simulink model "ECU_Arch"  (R2022b)
settings: Solver=FixedStepDiscrete  StartTime=0.0  StopTime=10.0  RelTol=1e-3
InitFcn:
  | mbd_mpc_consistency_checks(bdroot(gcs));
model workspace (MAT data in the model file):
  AlignmentIdRef = Simulink.Parameter
  AlignmentIdRef.Value = 0.3
  AlignmentIdRef.Description = 'The required IdRef ( which applaies a voltage vector) to aligne the rotor to detect the encoder or resolver offset'
  AlignmentIdRef.DataType = 'single'
  AlignmentIdRef.Min = 0.1
  AlignmentIdRef.Max = 100
  AlignmentIdRef.DocUnits = 'A'
  AlignmentIdRef.Complexity = 'real'
  AlignmentIdRef.Dimensions = [1 1]
  Alignment_ReqTime_sec = Simulink.Parameter
  Alignment_ReqTime_sec.Value = 3
  Alignment_ReqTime_sec.DataType = 'single'
  Alignment_ReqTime_sec.Min = 0
  Alignment_ReqTime_sec.Max = 20
  Alignment_ReqTime_sec.Complexity = 'real'
  Alignment_ReqTime_sec.Dimensions = [1 1]
  AliveCounterStartGD = Simulink.Signal
  AliveCounterStartGD.Description = 'Alive counter to check the length of the Init of GateDriver'
  AliveCounterStartGD.DataType = 'single'
  AliveCounterStartGD.Min = -1000000
  AliveCounterStartGD.Max = 1000000
  AliveCounterStartGD.DocUnits = '-'
  AliveCounterStartGD.Dimensions = -1
  AliveCounterStartGD.DimensionsMode = 'auto'
  AliveCounterStartGD.Complexity = 'auto'
  AliveCounterStartGD.SampleTime = -1
  AliveCounterStartGD.SamplingMode = 'auto'
  AliveCounterStartGD.InitialValue = '0'
  AngleChangeDir = Simulink.Parameter
  AngleChangeDir.Value = 1
  AngleChangeDir.Description = 'It can be used to change the direction of the postion signal, but by default = 1'
  AngleChangeDir.DataType = 'single'
  AngleChangeDir.Min = -1
  AngleChangeDir.Max = 1
  AngleChangeDir.Complexity = 'real'
  AngleChangeDir.Dimensions = [1 1]
  C_LST = 0.0001
  CtrlMode = Simulink.Parameter
  CtrlMode.Value = 1
  CtrlMode.DataType = 'single'
  CtrlMode.Min = 0
  CtrlMode.Max = 1
  CtrlMode.Complexity = 'real'
  CtrlMode.Dimensions = [1 1]
  DelayTimeAfterOL_sec = Simulink.Parameter
  DelayTimeAfterOL_sec.Value = 5
  DelayTimeAfterOL_sec.DataType = 'single'
  DelayTimeAfterOL_sec.Min = 0
  DelayTimeAfterOL_sec.Max = 100
  DelayTimeAfterOL_sec.Complexity = 'real'
  DelayTimeAfterOL_sec.Dimensions = [1 1]
  DisablePWM = Simulink.Parameter
  DisablePWM.Value = 0
  DisablePWM.Description = 'Disable the PWM during the Rotor Offset Calibration'
  DisablePWM.DataType = 'single'
  DisablePWM.Min = 0
  DisablePWM.Max = 1
  DisablePWM.Complexity = 'real'
  DisablePWM.Dimensions = [1 1]
  DisablePWM_Selector = Simulink.Parameter
  DisablePWM_Selector.Value = 0
  DisablePWM_Selector.Description = 'select either without or with Disable the PWM during the Rotor Offset Calibration'
  DisablePWM_Selector.DataType = 'uint8'
  DisablePWM_Selector.Min = 0
  DisablePWM_Selector.Max = 1
  DisablePWM_Selector.DocUnits = '-'
  DisablePWM_Selector.Complexity = 'real'
  DisablePWM_Selector.Dimensions = [1 1]
  ExecutionTimeFastLoop_FOC = Simulink.Parameter
  ExecutionTimeFastLoop_FOC.Value = 0
  ExecutionTimeFastLoop_FOC.Description = 'to measure the execution time of the subsystem'
  ExecutionTimeFastLoop_FOC.DataType = 'single'
  ExecutionTimeFastLoop_FOC.Min = 0
  ExecutionTimeFastLoop_FOC.Max = 1000000
  ExecutionTimeFastLoop_FOC.Complexity = 'real'
  ExecutionTimeFastLoop_FOC.Dimensions = [1 1]
  IDcFilterConst = Simulink.Parameter
  IDcFilterConst.Value = 0.001
  IDcFilterConst.Description = 'Time constant of the FIR IDc current filter '
  IDcFilterConst.DataType = 'single'
  IDcFilterConst.Min = 0
  IDcFilterConst.Max = 1
  IDcFilterConst.Complexity = 'real'
  IDcFilterConst.Dimensions = [1 1]
  IDcFilterSelector = Simulink.Parameter
  IDcFilterSelector.Value = 0
  IDcFilterSelector.Description = 'Switch to select one of the applied IDc current filter '
  IDcFilterSelector.DataType = 'uint16'
  IDcFilterSelector.Min = 0
  IDcFilterSelector.Max = 1
  IDcFilterSelector.Complexity = 'real'
  IDcFilterSelector.Dimensions = [1 1]
  IDcOvercurrent = Simulink.Parameter
  IDcOvercurrent.Value = 5
  IDcOvercurrent.Description = 'value of the overcurrent'
  IDcOvercurrent.DataType = 'single'
  IDcOvercurrent.Min = 0.1
  IDcOvercurrent.Max = 100
  IDcOvercurrent.DocUnits = 'A'
  IDcOvercurrent.Complexity = 'real'
  IDcOvercurrent.Dimensions = [1 1]
  IDcOvercurrentAlignment = Simulink.Parameter
  IDcOvercurrentAlignment.Value = 6
  IDcOvercurrentAlignment.Description = 'Idc overcurrent limit during rotor alignment to detect the encoder or resolver offset'
  IDcOvercurrentAlignment.DataType = 'single'
  IDcOvercurrentAlignment.Min = 0.1
  IDcOvercurrentAlignment.Max = 100
  IDcOvercurrentAlignment.DocUnits = 'A'
  IDcOvercurrentAlignment.Complexity = 'real'
  IDcOvercurrentAlignment.Dimensions = [1 1]
  IQ_REF = Simulink.Signal
  IQ_REF.Description = 'The reference iq'
  IQ_REF.DataType = 'single'
  IQ_REF.Min = -100
  IQ_REF.Max = 100
  IQ_REF.DocUnits = 'A'
  IQ_REF.Dimensions = -1
  IQ_REF.DimensionsMode = 'auto'
  IQ_REF.Complexity = 'real'
  IQ_REF.SampleTime = -1
  IQ_REF.SamplingMode = 'auto'
  IQ_REF.InitialValue = '0'
  IQ_REF_MAX = Simulink.Parameter
  IQ_REF_MAX.Value = 2.3
  IQ_REF_MAX.Description = 'Maximum allowed Iq current to limit the output of the speed controller'
  IQ_REF_MAX.DataType = 'single'
  IQ_REF_MAX.Min = -100
  IQ_REF_MAX.Max = 100
  IQ_REF_MAX.DocUnits = 'A'
  IQ_REF_MAX.Complexity = 'real'
  IQ_REF_MAX.Dimensions = [1 1]
  I_MAX = Simulink.Parameter
  I_MAX.Value = 20.625
  I_MAX.Description = 'Maximum current used for current measurement scaling calibration'
  I_MAX.DataType = 'single'
  I_MAX.Min = -100
  I_MAX.Max = 100
  I_MAX.DocUnits = 'A'
  I_MAX.Complexity = 'real'
  I_MAX.Dimensions = [1 1]
  KiId = Simulink.Parameter
  KiId.Value = 0.5
  KiId.Description = 'proportional parameter Kp of the ID-current controller'
  KiId.DataType = 'single'
  KiId.Min = 0
  KiId.Max = 1000
  KiId.Complexity = 'real'
  KiId.Dimensions = [1 1]
  KiIq = Simulink.Parameter
  KiIq.Value = 0.5
  KiIq.Description = 'proportional parameter Kp of the IQ-current controller'
  KiIq.DataType = 'single'
  KiIq.Min = 0
  KiIq.Max = 1000
  KiIq.Complexity = 'real'
  KiIq.Dimensions = [1 1]
  KiSpd = Simulink.Parameter
  KiSpd.Value = 1
  KiSpd.Description = 'propotinal factor of speed controller'
  KiSpd.DataType = 'single'
  KiSpd.Min = 0
  KiSpd.Max = 1000
  KiSpd.Complexity = 'real'
  KiSpd.Dimensions = [1 1]
  KiSpdOrg = Simulink.Parameter
  KiSpdOrg.Value = 2.2316799098e-05
  KiSpdOrg.Description = 'propotinal factor of speed controller'
  KiSpdOrg.DataType = 'single'
  KiSpdOrg.Min = 0
  KiSpdOrg.Max = 1000
  KiSpdOrg.Complexity = 'real'
  KiSpdOrg.Dimensions = [1 1]
  KpId = Simulink.Parameter
  KpId.Value = 0.3
  KpId.Description = 'proportional parameter Kp of the ID-current controller'
  KpId.DataType = 'single'
  KpId.Min = 0
  KpId.Max = 1000
  KpId.Complexity = 'real'
  KpId.Dimensions = [1 1]
  KpIq = Simulink.Parameter
  KpIq.Value = 0.3
  KpIq.Description = 'proportional parameter Kp of the IQ-current controller'
  KpIq.DataType = 'single'
  KpIq.Min = 0
  KpIq.Max = 1000
  KpIq.Complexity = 'real'
  KpIq.Dimensions = [1 1]
  KpSpd = Simulink.Parameter
  KpSpd.Value = 1.5
  KpSpd.Description = 'propotinal factor of speed controller'
  KpSpd.DataType = 'single'
  KpSpd.Min = 0
  KpSpd.Max = 1000
  KpSpd.Complexity = 'real'
  KpSpd.Dimensions = [1 1]
  KpSpdOrg = Simulink.Parameter
  KpSpdOrg.Value = 0.0142073155617
  KpSpdOrg.Description = 'propotinal factor of speed controller'
  KpSpdOrg.DataType = 'single'
  KpSpdOrg.Min = 0
  KpSpdOrg.Max = 1000
  KpSpdOrg.Complexity = 'real'
  KpSpdOrg.Dimensions = [1 1]
  Low_TQLimit_SpdCtrl = Simulink.Parameter
  Low_TQLimit_SpdCtrl.Value = -0.12
  Low_TQLimit_SpdCtrl.DataType = 'single'
  Low_TQLimit_SpdCtrl.Min = -10
  Low_TQLimit_SpdCtrl.Max = 0
  Low_TQLimit_SpdCtrl.Complexity = 'real'
  Low_TQLimit_SpdCtrl.Dimensions = [1 1]
  Low_TQLimit_TqCtrl = Simulink.Parameter
  Low_TQLimit_TqCtrl.Value = -0.04
  Low_TQLimit_TqCtrl.DataType = 'single'
  Low_TQLimit_TqCtrl.Min = -10
  Low_TQLimit_TqCtrl.Max = 0
  Low_TQLimit_TqCtrl.Complexity = 'real'
  Low_TQLimit_TqCtrl.Dimensions = [1 1]
  MaxSpdLimit = Simulink.Parameter
  MaxSpdLimit.Value = 199
  MaxSpdLimit.Description = 'Maximum Allowed Speed'
  MaxSpdLimit.DataType = 'single'
  MaxSpdLimit.Min = -524
  MaxSpdLimit.Max = 524
  MaxSpdLimit.DocUnits = 'rad/sec'
  MaxSpdLimit.Complexity = 'real'
  MaxSpdLimit.Dimensions = [1 1]
  Nmax = Simulink.Parameter
  Nmax.Value = 6000
  Nmax.Description = 'polpair'
  Nmax.DataType = 'int32'
  Nmax.Min = 1
  Nmax.Max = 20000
  Nmax.DocUnits = '-'
  Nmax.Complexity = 'real'
  Nmax.Dimensions = [1 1]
  OL_IDcOvercurrent = Simulink.Parameter
  OL_IDcOvercurrent.Value = 5.5
  OL_IDcOvercurrent.DataType = 'single'
  OL_IDcOvercurrent.Min = 0
  OL_IDcOvercurrent.Max = 7
  OL_IDcOvercurrent.Complexity = 'real'
  OL_IDcOvercurrent.Dimensions = [1 1]
  OL_ReqTime_sec = Simulink.Parameter
  OL_ReqTime_sec.Value = 1
  OL_ReqTime_sec.DataType = 'single'
  OL_ReqTime_sec.Min = 0
  OL_ReqTime_sec.Max = 20
  OL_ReqTime_sec.Complexity = 'real'
  OL_ReqTime_sec.Dimensions = [1 1]
  OffsetSelector = Simulink.Parameter
  OffsetSelector.Value = 0
  OffsetSelector.Description = 'switch to select the finial rotor offset either add to the actual rotor position or substract from the actual rotor position'
  OffsetSelector.DataType = 'uint8'
  OffsetSelector.Min = 0
  OffsetSelector.Max = 1
  OffsetSelector.Complexity = 'real'
  OffsetSelector.Dimensions = [1 1]
  PISpdControllerSelector = Simulink.Parameter
  PISpdControllerSelector.Value = 0
  PISpdControllerSelector.Description = 'selector to test the correct PI speed controller'
  PISpdControllerSelector.DataType = 'uint8'
  PISpdControllerSelector.Min = 0
  PISpdControllerSelector.Max = 1
  PISpdControllerSelector.Complexity = 'real'
  PISpdControllerSelector.Dimensions = [1 1]
  PMflux = Simulink.Parameter
  PMflux.Value = 0.0064
  PMflux.DataType = 'single'
  PMflux.Min = 0
  PMflux.Max = 10
  PMflux.Complexity = 'real'
  PMflux.Dimensions = [1 1]
  PP = Simulink.Parameter
  PP.Value = 4
  PP.Description = 'polpair'
  PP.DataType = 'int32'
  PP.Min = 1
  PP.Max = 10
  PP.DocUnits = '-'
  PP.Complexity = 'real'
  PP.Dimensions = [1 1]
  PWMDutyCycle_A = Simulink.Signal
  PWMDutyCycle_A.Description = 'Input of the PWM Phase A '
  PWMDutyCycle_A.DataType = 'single'
  PWMDutyCycle_A.Min = -100
  PWMDutyCycle_A.Max = 100
  PWMDutyCycle_A.DocUnits = '-'
  PWMDutyCycle_A.Dimensions = -1
  PWMDutyCycle_A.DimensionsMode = 'auto'
  PWMDutyCycle_A.Complexity = 'real'
  PWMDutyCycle_A.SampleTime = -1
  PWMDutyCycle_A.SamplingMode = 'auto'
  PWMDutyCycle_A.InitialValue = '0'
  PWMDutyCycle_B = Simulink.Signal
  PWMDutyCycle_B.Description = 'Input of the PWM Phase B '
  PWMDutyCycle_B.DataType = 'single'
  PWMDutyCycle_B.Min = -100
  PWMDutyCycle_B.Max = 100
  PWMDutyCycle_B.DocUnits = '-'
  PWMDutyCycle_B.Dimensions = -1
  PWMDutyCycle_B.DimensionsMode = 'auto'
  PWMDutyCycle_B.Complexity = 'real'
  PWMDutyCycle_B.SampleTime = -1
  PWMDutyCycle_B.SamplingMode = 'auto'
  PWMDutyCycle_B.InitialValue = '0'
  PWMDutyCycle_C = Simulink.Signal
  PWMDutyCycle_C.Description = 'Input of the PWM Phase C '
  PWMDutyCycle_C.DataType = 'single'
  PWMDutyCycle_C.Min = -100
  PWMDutyCycle_C.Max = 100
  PWMDutyCycle_C.DocUnits = '-'
  PWMDutyCycle_C.Dimensions = -1
  PWMDutyCycle_C.DimensionsMode = 'auto'
  PWMDutyCycle_C.Complexity = 'real'
  PWMDutyCycle_C.SampleTime = -1
  PWMDutyCycle_C.SamplingMode = 'auto'
  PWMDutyCycle_C.InitialValue = '0'
  PhA_Offset = Simulink.Parameter
  PhA_Offset.Value = 20.625
  PhA_Offset.Description = 'Offset current value of phase A, which used for current calibration'
  PhA_Offset.DataType = 'single'
  PhA_Offset.Min = -100
  PhA_Offset.Max = 100
  PhA_Offset.DocUnits = 'A'
  PhA_Offset.Complexity = 'real'
  PhA_Offset.Dimensions = [1 1]
  PhB_Offset = Simulink.Parameter
  PhB_Offset.Value = 20.625
  PhB_Offset.Description = 'Offset current value of phase B, which used for current calibration'
  PhB_Offset.DataType = 'single'
  PhB_Offset.Min = -100
  PhB_Offset.Max = 100
  PhB_Offset.DocUnits = 'A'
  PhB_Offset.Complexity = 'real'
  PhB_Offset.Dimensions = [1 1]
  RotorOffsetMotor1_Selector = Simulink.Parameter
  RotorOffsetMotor1_Selector.Value = 1
  RotorOffsetMotor1_Selector.Description = 'Feedback when the rotor offset of motor1 is completed '
  RotorOffsetMotor1_Selector.DataType = 'single'
  RotorOffsetMotor1_Selector.Min = 0
  RotorOffsetMotor1_Selector.Max = 1
  RotorOffsetMotor1_Selector.DocUnits = '-'
  RotorOffsetMotor1_Selector.Complexity = 'real'
  RotorOffsetMotor1_Selector.Dimensions = [1 1]
  RotorOffsetMotor2_Selector = Simulink.Parameter
  RotorOffsetMotor2_Selector.Value = 1
  RotorOffsetMotor2_Selector.Description = 'Feedback when the rotor offset of motor2 is completed '
  RotorOffsetMotor2_Selector.DataType = 'single'
  RotorOffsetMotor2_Selector.Min = 0
  RotorOffsetMotor2_Selector.Max = 1
  RotorOffsetMotor2_Selector.DocUnits = '-'
  RotorOffsetMotor2_Selector.Complexity = 'real'
  RotorOffsetMotor2_Selector.Dimensions = [1 1]
  SPEED_CMD = Simulink.Parameter
  SPEED_CMD.Value = 500
  SPEED_CMD.Description = 'Reference speed in rpm'
  SPEED_CMD.DataType = 'single'
  SPEED_CMD.Min = -2200
  SPEED_CMD.Max = 2200
  SPEED_CMD.Complexity = 'real'
  SPEED_CMD.Dimensions = [1 1]
  SPEED_DOWN_INC = Simulink.Parameter
  SPEED_DOWN_INC.Value = 50
  SPEED_DOWN_INC.Description = 'Gain used to decrease the reference speed (SPEED_CMD)using push botton on the MPC5744P board '
  SPEED_DOWN_INC.DataType = 'single'
  SPEED_DOWN_INC.Min = -1000
  SPEED_DOWN_INC.Max = 1000
  SPEED_DOWN_INC.Complexity = 'real'
  SPEED_DOWN_INC.Dimensions = [1 1]
  SPEED_LOOP_CNTR = Simulink.Parameter
  SPEED_LOOP_CNTR.Value = 10
  SPEED_LOOP_CNTR.Description = 'speed loop counter, which used to determine who many current loops are over to recall the speed loop  '
  SPEED_LOOP_CNTR.DataType = 'single'
  SPEED_LOOP_CNTR.Min = -1000
  SPEED_LOOP_CNTR.Max = 1000
  SPEED_LOOP_CNTR.Complexity = 'real'
  SPEED_LOOP_CNTR.Dimensions = [1 1]
  SPEED_UP_INC = Simulink.Parameter
  SPEED_UP_INC.Value = 50
  SPEED_UP_INC.Description = 'Gain used to decrease the reference speed (SPEED_CMD)using push botton on the MPC5744P board '
  SPEED_UP_INC.DataType = 'single'
  SPEED_UP_INC.Min = -1000
  SPEED_UP_INC.Max = 1000
  SPEED_UP_INC.Complexity = 'real'
  SPEED_UP_INC.Dimensions = [1 1]
  S_LST = 0.001
  SpdChangeDir = Simulink.Parameter
  SpdChangeDir.Value = 1
  SpdChangeDir.Description = 'It can be used to change the direction of the speed signal, but by default = 1'
  SpdChangeDir.DataType = 'single'
  SpdChangeDir.Min = -1
  SpdChangeDir.Max = 1
  SpdChangeDir.Complexity = 'real'
  SpdChangeDir.Dimensions = [1 1]
  SpdDecreasingStep = Simulink.Parameter
  SpdDecreasingStep.Value = 0.01
  SpdDecreasingStep.DataType = 'single'
  SpdDecreasingStep.Min = 0
  SpdDecreasingStep.Max = 100
  SpdDecreasingStep.Complexity = 'real'
  SpdDecreasingStep.Dimensions = [1 1]
  SpdFilterConst = Simulink.Parameter
  SpdFilterConst.Value = 0.0005
  SpdFilterConst.Description = 'Time constant of the FIR speed filter '
  SpdFilterConst.DataType = 'single'
  SpdFilterConst.Min = 0
  SpdFilterConst.Max = 1
  SpdFilterConst.Complexity = 'real'
  SpdFilterConst.Dimensions = [1 1]
  SpeedAct = Simulink.Signal
  SpeedAct.Description = 'The measured actual speed in rad/sec'
  SpeedAct.DataType = 'single'
  SpeedAct.Min = -200000
  SpeedAct.Max = 20000
  SpeedAct.DocUnits = 'rad/sec'
  SpeedAct.Dimensions = -1
  SpeedAct.DimensionsMode = 'auto'
  SpeedAct.Complexity = 'real'
  SpeedAct.SampleTime = -1
  SpeedAct.SamplingMode = 'auto'
  SpeedAct.InitialValue = '0'
  SpeedActRpm = Simulink.Signal
  SpeedActRpm.Description = 'The measured actual speed in rpm'
  SpeedActRpm.DataType = 'single'
  SpeedActRpm.Min = -20000
  SpeedActRpm.Max = 20000
  SpeedActRpm.DocUnits = 'rpm'
  SpeedActRpm.Dimensions = -1
  SpeedActRpm.DimensionsMode = 'auto'
  SpeedActRpm.Complexity = 'real'
  SpeedActRpm.SampleTime = -1
  SpeedActRpm.SamplingMode = 'auto'
  SpeedActRpm.InitialValue = '0'
  SpeedCmd = Simulink.Signal
  SpeedCmd.Description = 'The speed command in rpm'
  SpeedCmd.DataType = 'single'
  SpeedCmd.Min = -20000
  SpeedCmd.Max = 20000
  SpeedCmd.DocUnits = 'rad/sec'
  SpeedCmd.Dimensions = -1
  SpeedCmd.DimensionsMode = 'auto'
  SpeedCmd.Complexity = 'real'
  SpeedCmd.SampleTime = -1
  SpeedCmd.SamplingMode = 'auto'
  SpeedCmd.InitialValue = '0'
  SpeedRef = Simulink.Signal
  SpeedRef.Description = 'The reference speed in rad/sec after filtered SPEED_Cmd'
  SpeedRef.DataType = 'single'
  SpeedRef.Min = -2000
  SpeedRef.Max = 2000
  SpeedRef.DocUnits = 'rad/sec'
  SpeedRef.Dimensions = -1
  SpeedRef.DimensionsMode = 'auto'
  SpeedRef.Complexity = 'real'
  SpeedRef.SampleTime = -1
  SpeedRef.SamplingMode = 'auto'
  SpeedRef.InitialValue = '0'
  SpeedThresholdOvercurrent = Simulink.Parameter
  SpeedThresholdOvercurrent.Value = 0
  SpeedThresholdOvercurrent.Description = 'This is speed threshold in rad/sec, which is used to switch the another IDc overcurrent value to meet the high current of Teknic M-2310P-LN-04K during the rotor alignment'
  SpeedThresholdOvercurrent.DataType = 'single'
  SpeedThresholdOvercurrent.Min = 0
  SpeedThresholdOvercurrent.Max = 40
  SpeedThresholdOvercurrent.Complexity = 'real'
  SpeedThresholdOvercurrent.Dimensions = [1 1]
  ThetaOffsetIncEncoder = Simulink.Signal
  ThetaOffsetIncEncoder.Description = 'The detected rotor offset of the incremental encoder'
  ThetaOffsetIncEncoder.DataType = 'single'
  ThetaOffsetIncEncoder.Min = -1000
  ThetaOffsetIncEncoder.Max = 1000
  ThetaOffsetIncEncoder.DocUnits = 'rad'
  ThetaOffsetIncEncoder.Dimensions = -1
  ThetaOffsetIncEncoder.DimensionsMode = 'auto'
  ThetaOffsetIncEncoder.Complexity = 'real'
  ThetaOffsetIncEncoder.SampleTime = -1
  ThetaOffsetIncEncoder.SamplingMode = 'auto'
  ThetaOffsetIncEncoder.InitialValue = '0'
  Torque_Ref = Simulink.Signal
  Torque_Ref.Description = 'The reference torque'
  Torque_Ref.DataType = 'single'
  Torque_Ref.Min = -100
  Torque_Ref.Max = 100
  Torque_Ref.DocUnits = 'Nm'
  Torque_Ref.Dimensions = -1
  Torque_Ref.DimensionsMode = 'auto'
  Torque_Ref.Complexity = 'auto'
  Torque_Ref.SampleTime = -1
  Torque_Ref.SamplingMode = 'auto'
  Torque_Ref.InitialValue = '0'
  TqCtrlRef = Simulink.Parameter
  TqCtrlRef.Value = 0.03
  TqCtrlRef.Description = 'Reference Torque'
  TqCtrlRef.DataType = 'single'
  TqCtrlRef.Min = -3
  TqCtrlRef.Max = 3
  TqCtrlRef.DocUnits = 'Nm'
  TqCtrlRef.Complexity = 'real'
  TqCtrlRef.Dimensions = [1 1]
  TqCtrlSwitch = Simulink.Parameter
  TqCtrlSwitch.Value = 0
  TqCtrlSwitch.Description = 'Switch to select Speed Control "0" or Torque Control "1"'
  TqCtrlSwitch.DataType = 'boolean'
  TqCtrlSwitch.Min = 0
  TqCtrlSwitch.Max = 1
  TqCtrlSwitch.Complexity = 'real'
  TqCtrlSwitch.Dimensions = [1 1]
  TqDecreasingStep = Simulink.Parameter
  TqDecreasingStep.Value = 3e-06
  TqDecreasingStep.DataType = 'single'
  TqDecreasingStep.Min = 0
  TqDecreasingStep.Max = 100
  TqDecreasingStep.Complexity = 'real'
  TqDecreasingStep.Dimensions = [1 1]
  TqFilterConst = Simulink.Parameter
  TqFilterConst.Value = 0.001
  TqFilterConst.Description = 'Time constant of the FIR torque filter '
  TqFilterConst.DataType = 'single'
  TqFilterConst.Min = 0
  TqFilterConst.Max = 1
  TqFilterConst.DocUnits = '-'
  TqFilterConst.Complexity = 'real'
  TqFilterConst.Dimensions = [1 1]
  TrgTime = Simulink.Parameter
  TrgTime.Value = 10000
  TrgTime.DataType = 'single'
  TrgTime.Min = 0
  TrgTime.Max = 10000000
  TrgTime.Complexity = 'real'
  TrgTime.Dimensions = [1 1]
  UAlpha = Simulink.Signal
  UAlpha.Description = 'voltage on alpha axis related to the Alpha-Beta coordination system'
  UAlpha.DataType = 'single'
  UAlpha.Min = -500
  UAlpha.Max = 500
  UAlpha.DocUnits = 'V'
  UAlpha.Dimensions = -1
  UAlpha.DimensionsMode = 'auto'
  UAlpha.Complexity = 'real'
  UAlpha.SampleTime = -1
  UAlpha.SamplingMode = 'auto'
  UAlpha.InitialValue = '0'
  UBeta = Simulink.Signal
  UBeta.Description = 'voltage on beta axis related to the Alpha-Beta coordination system'
  UBeta.DataType = 'single'
  UBeta.Min = -500
  UBeta.Max = 500
  UBeta.DocUnits = 'V'
  UBeta.Dimensions = -1
  UBeta.DimensionsMode = 'auto'
  UBeta.Complexity = 'real'
  UBeta.SampleTime = -1
  UBeta.SamplingMode = 'auto'
  UBeta.InitialValue = '0'
  UP_TQLimit_SpdCtrl = Simulink.Parameter
  UP_TQLimit_SpdCtrl.Value = 0.12
  UP_TQLimit_SpdCtrl.DataType = 'single'
  UP_TQLimit_SpdCtrl.Min = 0
  UP_TQLimit_SpdCtrl.Max = 10
  UP_TQLimit_SpdCtrl.Complexity = 'real'
  UP_TQLimit_SpdCtrl.Dimensions = [1 1]
  UP_TQLimit_TqCtrl = Simulink.Parameter
  UP_TQLimit_TqCtrl.Value = 0.04
  UP_TQLimit_TqCtrl.DataType = 'single'
  UP_TQLimit_TqCtrl.Min = 0
  UP_TQLimit_TqCtrl.Max = 10
  UP_TQLimit_TqCtrl.Complexity = 'real'
  UP_TQLimit_TqCtrl.Dimensions = [1 1]
  VDC_OVERVOLTAGE = Simulink.Parameter
  VDC_OVERVOLTAGE.Value = 18
  VDC_OVERVOLTAGE.Description = 'Overvoltage protection  '
  VDC_OVERVOLTAGE.DataType = 'single'
  VDC_OVERVOLTAGE.Min = -1000
  VDC_OVERVOLTAGE.Max = 1000
  VDC_OVERVOLTAGE.Complexity = 'real'
  VDC_OVERVOLTAGE.Dimensions = [1 1]
  VDC_UNDERVOLTAGE = Simulink.Parameter
  VDC_UNDERVOLTAGE.Value = 8
  VDC_UNDERVOLTAGE.Description = 'Undervoltage protection '
  VDC_UNDERVOLTAGE.DataType = 'single'
  VDC_UNDERVOLTAGE.Min = -1000
  VDC_UNDERVOLTAGE.Max = 1000
  VDC_UNDERVOLTAGE.Complexity = 'real'
  VDC_UNDERVOLTAGE.Dimensions = [1 1]
  WaitingTimeAfterAlignment_sec = Simulink.Parameter
  WaitingTimeAfterAlignment_sec.Value = 5
  WaitingTimeAfterAlignment_sec.DataType = 'single'
  WaitingTimeAfterAlignment_sec.Min = 0
  WaitingTimeAfterAlignment_sec.Max = 100
  WaitingTimeAfterAlignment_sec.Complexity = 'real'
  WaitingTimeAfterAlignment_sec.Dimensions = [1 1]
undefined symbols (not defined in the file): LQFP
libraries: nesl_utility x5, simulink x2, mbd_mpc574x_ec_toolbox x1
settings Model: Creator=MAAM  LastModifiedBy=MAAM
settings DataIOCC: ExternalInput=off  InitialState=off  SaveOutput=off  SignalLogging=off  SaveTime=off
settings OptimizationCC: DefaultParameterBehavior=Inlined  EnhancedBackFolding=on  PassReuseOutputArgsAs=Individual arguments  ZeroExternalMemoryAtStartup=off  ZeroInternalMemoryAtStartup=off  OptimizeBlockOrder=speed  DifferentSizesBufferReuse=on  OptimizationCustomize=off  EfficientTunableParamExpr=on
settings DebuggingCC: InheritedTsInSrcMsg=none  ParameterTunabilityLossMsg=error
settings HardwareCC: ProdBitPerPointer=32  ProdBitPerSizeT=32  ProdBitPerPtrDiffT=32  ProdLargestAtomicInteger=Long  ProdLargestAtomicFloat=Double  ProdEndianess=BigEndian  ProdWordSize=32  ProdHWDeviceType=Motorola PowerPC
settings SFSimCC: MATLABDynamicMemAlloc=off
settings RTWCC: Description=Model Based Design Toolbox MPC57xx Code Generation Target  SystemTargetFile=mbd_mpc574x.tlc  MakeCommand=mbd_mpc574x_make_rtw  TemplateMakefile=mbd_mpc574x.tmf
settings CodeAppCC: ForceParamTrailComments=on  IgnoreCustomStorageClasses=off  OperatorAnnotations=on  SimulinkDataObjDesc=on  SFDataObjDesc=on  InsertBlockDesc=on
settings STFCustomTargetCC: TargetLangStandard=C99 (ISO)  MultiwordLength=256  CombineOutputUpdateFcns=on  ERTCustomFileBanners=on  SupportContinuousTime=off  SupportNonInlinedSFcns=off  RemoveResetFunc=on  MATLABClassNameForMDSCustomization=Simulink.SoftwareTarget.ERTCustomization  SystemTargetFile=mbd_mpc574x.tlc
settings ERTTargetCC: TargetLangStandard=C99 (ISO)  ParMdlRefBuildCompliant=off  CompOptLevelCompliant=off  ConcurrentExecutionCompliant=off  ModelStepFunctionPrototypeControlCompliant=off  CPPClassGenCompliant=off  UseToolchainInfoCompliant=off  InlinedParameterPlacement=NonHierarchical  ERTCustomFileTemplate=example_file_process.tlc

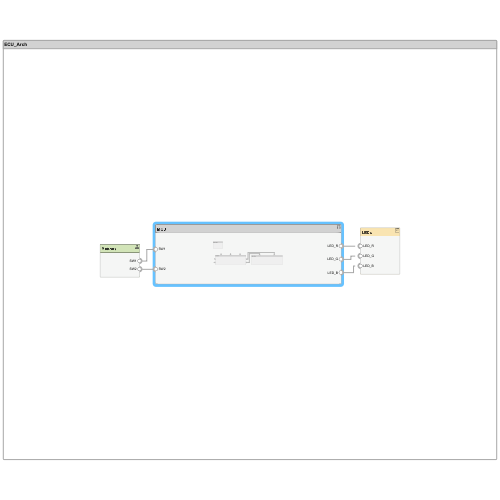
[thumbnail: Simulink's stored preview of the top-level diagram]
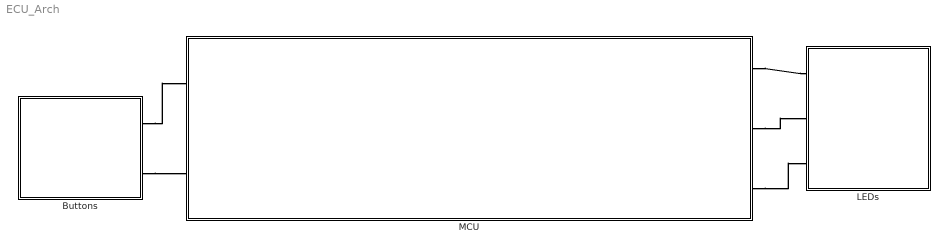
== system ECU_Arch ==
  Buttons : Subsystem
      settings: PortSchema="{\"entries\":[{\"content\":{\"headerSize\":26,\"margin\":15,\"minimumSpacing\":25,\"sides\":[{\"content\":{\"connectorIds\":[]},\"type\":\"ConnectorPlacement.EquallySpacedRectSide\",\"uuid\":\"beb8852d-a87e-4145-8686-8a29382e5b86\"},{\"content\":{\"connectorIds\":[\"RConn1\",\"RConn2\"],\"side\":\"RIGHT\"},\"type\":\"ConnectorPlacement.EquallySpacedRectSide\",\"uuid\":\"d0e85422-4355-4f6a-9555-942e64611473\"},{\"content\":{\"connectorIds\":[],\"side\":\"TOP\"},\"type\":\"ConnectorPlacement.EquallySpacedRectSide\",\"uuid\":\"a53edc1f-d2b9-4f5a-94ce-d565a9112b3f\"}]},\"type\":\"ConnectorPlacement.EquallySpacedConnector\",\"uuid\":\"8a26cbf3-c9e2-4af5-bc86-3460ae1a178f\"}],\"packageUris\":[\"http://schema.mathworks.com/mf0/Connector/R2020b\"],\"version\":\"1.0\"}"
  LEDs : Subsystem
      settings: PortSchema="{\"entries\":[{\"content\":{\"headerSize\":26,\"margin\":15,\"minimumSpacing\":25,\"sides\":[{\"content\":{\"connectorIds\":[\"LConn1\",\"LConn2\",\"LConn3\"]},\"type\":\"ConnectorPlacement.EquallySpacedRectSide\",\"uuid\":\"beb8852d-a87e-4145-8686-8a29382e5b86\"},{\"content\":{\"connectorIds\":[],\"side\":\"RIGHT\"},\"type\":\"ConnectorPlacement.EquallySpacedRectSide\",\"uuid\":\"d0e85422-4355-4f6a-9555-942e64611473\"},{\"content\":{\"connectorIds\":[],\"side\":\"TOP\"},\"type\":\"ConnectorPlacement.EquallySpacedRectSide\",\"uuid\":\"a53edc1f-d2b9-4f5a-94ce-d565a9112b3f\"}]},\"type\":\"ConnectorPlacement.EquallySpacedConnector\",\"uuid\":\"8a26cbf3-c9e2-4af5-bc86-3460ae1a178f\"}],\"packageUris\":[\"http://schema.mathworks.com/mf0/Connector/R2020b\"],\"version\":\"1.0\"}"
  MCU : Subsystem
      settings: PortSchema="{\"entries\":[{\"content\":{\"headerSize\":26,\"margin\":15,\"minimumSpacing\":25,\"sides\":[{\"content\":{\"connectorIds\":[\"LConn1\",\"LConn2\"]},\"type\":\"ConnectorPlacement.EquallySpacedRectSide\",\"uuid\":\"9fafbac4-d9ff-4bef-9686-25ce946f922a\"},{\"content\":{\"connectorIds\":[\"RConn1\",\"RConn2\",\"RConn3\"],\"side\":\"RIGHT\"},\"type\":\"ConnectorPlacement.EquallySpacedRectSide\",\"uuid\":\"64958763-52cc-4c3d-9da1-de7e7fca94ff\"},{\"content\":{\"connectorIds\":[],\"side\":\"TOP\"},\"type\":\"ConnectorPlacement.EquallySpacedRectSide\",\"uuid\":\"29c78429-a934-4b6b-906c-5a3963e1854a\"},{\"content\":{\"connectorIds\":[],\"side\":\"BOTTOM\"},\"type\":\"ConnectorPlacement.EquallySpacedRectSide\",\"uuid\":\"f9f9d59b-2161-4ff7-aea9-ea3466aa3e9c\"}]},\"type\":\"ConnectorPlacement.EquallySpacedConnector\",\"uuid\":\"b6b0d473-12c9-4a38-8dee-bffc8352e44f\"}],\"packageUris\":[\"http://schema.mathworks.com/mf0/Connector/R2020b\"],\"version\":\"1.0\"}"
  connections:
  MCU/RConn1 -- LEDs/LConn1
  Buttons/RConn1 -- MCU/LConn1
  Buttons/RConn2 -- MCU/LConn2
  MCU/RConn2 -- LEDs/LConn2
  MCU/RConn3 -- LEDs/LConn3

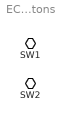
== system ECU_Arch/Buttons ==
  SW1 : PMIOPort  Side=Right
  SW2 : PMIOPort  Port=2  Side=Right

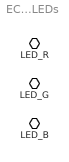
== system ECU_Arch/LEDs ==
  LED_R : PMIOPort  Side=Left
  LED_G : PMIOPort  Port=2  Side=Left
  LED_B : PMIOPort  Port=3  Side=Left

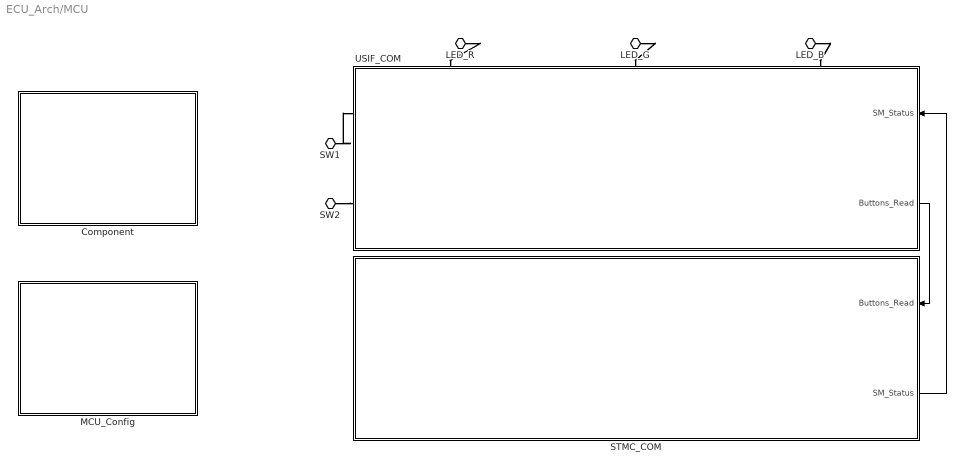
== system ECU_Arch/MCU ==
  Component : Subsystem
      settings: PortSchema="{\"entries\":[{\"content\":{\"headerSize\":26,\"margin\":15,\"minimumSpacing\":25,\"sides\":[{\"content\":{\"connectorIds\":[]},\"type\":\"ConnectorPlacement.EquallySpacedRectSide\",\"uuid\":\"86444d43-2102-435b-8a2b-2b030df31f7f\"},{\"content\":{\"connectorIds\":[],\"side\":\"RIGHT\"},\"type\":\"ConnectorPlacement.EquallySpacedRectSide\",\"uuid\":\"c9affe92-4cbe-435b-b672-be3201d83085\"},{\"content\":{\"connectorIds\":[],\"side\":\"TOP\"},\"type\":\"ConnectorPlacement.EquallySpacedRectSide\",\"uuid\":\"e6c64d0d-1c2e-4e7d-8b2e-cc6685d12efc\"}]},\"type\":\"ConnectorPlacement.EquallySpacedConnector\",\"uuid\":\"f562d7e9-72f8-4f82-93b3-f0475cfb8281\"}],\"packageUris\":[\"http://schema.mathworks.com/mf0/Connector/R2020b\"],\"version\":\"1.0\"}"
  MCU_Config : Subsystem
      settings: PortSchema="{\"entries\":[{\"content\":{\"headerSize\":26,\"margin\":15,\"minimumSpacing\":25,\"sides\":[{\"content\":{\"connectorIds\":[]},\"type\":\"ConnectorPlacement.EquallySpacedRectSide\",\"uuid\":\"9e3c9234-344f-41fb-9145-1ecb76f9604b\"},{\"content\":{\"connectorIds\":[],\"side\":\"RIGHT\"},\"type\":\"ConnectorPlacement.EquallySpacedRectSide\",\"uuid\":\"91314b46-0148-4d0b-8df6-e1be712fb317\"},{\"content\":{\"connectorIds\":[],\"side\":\"TOP\"},\"type\":\"ConnectorPlacement.EquallySpacedRectSide\",\"uuid\":\"6d51069f-a7df-430f-ba3a-6b16d510f018\"}]},\"type\":\"ConnectorPlacement.EquallySpacedConnector\",\"uuid\":\"067f1f1b-f809-4f0e-9eeb-c5481468f53e\"}],\"packageUris\":[\"http://schema.mathworks.com/mf0/Connector/R2020b\"],\"version\":\"1.0\"}"
  STMC_COM : Subsystem
      settings: PortSchema="{\"entries\":[{\"content\":{\"headerSize\":26,\"margin\":15,\"minimumSpacing\":25,\"sides\":[{\"content\":{\"connectorIds\":[]},\"type\":\"ConnectorPlacement.EquallySpacedRectSide\",\"uuid\":\"9e3c9234-344f-41fb-9145-1ecb76f9604b\"},{\"content\":{\"connectorIds\":[\"In1\",\"Out1\"],\"side\":\"RIGHT\"},\"type\":\"ConnectorPlacement.EquallySpacedRectSide\",\"uuid\":\"91314b46-0148-4d0b-8df6-e1be712fb317\"},{\"content\":{\"connectorIds\":[],\"side\":\"TOP\"},\"type\":\"ConnectorPlacement.EquallySpacedRectSide\",\"uuid\":\"6d51069f-a7df-430f-ba3a-6b16d510f018\"}]},\"type\":\"ConnectorPlacement.EquallySpacedConnector\",\"uuid\":\"067f1f1b-f809-4f0e-9eeb-c5481468f53e\"}],\"packageUris\":[\"http://schema.mathworks.com/mf0/Connector/R2020b\"],\"version\":\"1.0\"}"
  USIF_COM : Subsystem
      settings: PortSchema="{\"entries\":[{\"content\":{\"headerSize\":26,\"margin\":15,\"minimumSpacing\":25,\"sides\":[{\"content\":{\"connectorIds\":[\"LConn1\",\"LConn2\"]},\"type\":\"ConnectorPlacement.EquallySpacedRectSide\",\"uuid\":\"86444d43-2102-435b-8a2b-2b030df31f7f\"},{\"content\":{\"connectorIds\":[\"In1\",\"Out1\"],\"side\":\"RIGHT\"},\"type\":\"ConnectorPlacement.EquallySpacedRectSide\",\"uuid\":\"c9affe92-4cbe-435b-b672-be3201d83085\"},{\"content\":{\"connectorIds\":[\"LConn3\",\"LConn4\",\"LConn5\"],\"side\":\"TOP\"},\"type\":\"ConnectorPlacement.EquallySpacedRectSide\",\"uuid\":\"e6c64d0d-1c2e-4e7d-8b2e-cc6685d12efc\"}]},\"type\":\"ConnectorPlacement.EquallySpacedConnector\",\"uuid\":\"f562d7e9-72f8-4f82-93b3-f0475cfb8281\"}],\"packageUris\":[\"http://schema.mathworks.com/mf0/Connector/R2020b\"],\"version\":\"1.0\"}"
  SW1 : PMIOPort  Side=Left
  SW2 : PMIOPort  Port=2  Side=Left
  LED_R : PMIOPort  Port=3  Side=Right
  LED_G : PMIOPort  Port=4  Side=Right
  LED_B : PMIOPort  Port=5  Side=Right
  wires:
  USIF_COM/1(Buttons_Read) -> STMC_COM/1(Buttons_Read)
  STMC_COM/1(SM_Status) -> USIF_COM/1(SM_Status)
  connections:
  LED_R/RConn1 -- USIF_COM/LConn3
  LED_G/RConn1 -- USIF_COM/LConn4
  LED_B/RConn1 -- USIF_COM/LConn5
  SW1/RConn1 -- USIF_COM/LConn1
  SW2/RConn1 -- USIF_COM/LConn2

== system ECU_Arch/MCU/Component ==

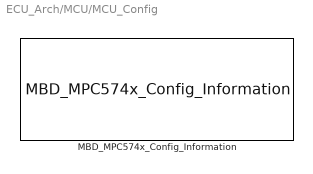
== system ECU_Arch/MCU/MCU_Config ==
  MBD_MPC574x_Config_Information : mbd_mpc574x_ec_toolbox/MBD_MPC574x_Config_Information  Priority=1  disp_str=|  config_params=[]  mcu_target_name=MPC5744P  mcu_target_package=144-LQFP  mcu_target_sram_size=384KB  mcu_system_clock_freq=200  mcu_xtal_freq=40  mcu_step_timer=PIT Channel 0  mcu_step_priority=1  ds_import_enable=on  target_compiler=S32 Design Studio  target_memory=FLASH  s32ds_target_compile_opts=-g3 -mbig -mvle -O1 -mregnames -mlsp -specs=ewl_c9x.specs -mhard-float -Wall -c -std=c99 -fdata-sections -ffunction-sections -funsigned-char -fmessage-length=0 -nostdinc -fno-jump-tables -DTURN_ON_CPU0  s32ds_target_assemble_opts=-g3 -mbig -mvle -mregnames -O1 -DTURN_ON_CPU0 -mhard-float  s32ds_target_link_opts=-Xlinker -gc-sections  s32ds_target_default_lcf=on  s32ds_target_user_lcf=MPC5744P_flash.ld  ghs_target_compile_opts=-G -filetype.c  ghs_target_assemble_opts=-G -filetype.assembly  ghs_target_default_lcf=on  ghs_target_user_lcf=MPC5744P_flash.ld  diab_target_compile_opts=-@E+err.log -c -g -Xenum-is-best -Xlint -Xnested-interrupts -Xdebug-local-cie -Xclib-optim-off -Xc-new  diab_target_assemble_opts=-@E+err.log -l -g  diab_target_link_opts=-@E+err.log -Ws -m6 -lc -lm  diab_target_default_lcf=on  diab_target_user_lcf=MPC5744P_flash.dld  pil_download_enable=off  rbl_download_enable=on  rbl_start_delay=5000  rbl_restart_request=on  rbl_com_port=Custom  rbl_com_port_custom=COM10  pil_download_rate=115200  pil_interface=Serial 0  pil_rx=PTB3: [LIN0_RX | LIN 0 Receive Pin]  pil_tx=PTB2: [LIN0_TX | LINFlexD 0 Transmit Pin]  rbl_def_password=on  rbl_password=0xFEEDFACECAFEBEEF  rbl_manual_len_size=off  rbl_start_address=0  rbl_code_size=0  ADC_PcrCheckEnDis=on  FlexPWM_PcrCheckEnDis=on  CTU_PcrCheckEnDis=on  SWG_PcrCheckEnDis=on  eTimer_PcrCheckEnDis=off  EQADC_PcrCheckEnDis=on  eMIOS_PcrCheckEnDis=on  FlexCAN_PcrCheckEnDis=on  I2C_PcrCheckEnDis=on  MCAN_PcrCheckEnDis=on  SPI_PcrCheckEnDis=on  UART_PcrCheckEnDis=on  GPIO_OutputPcrCheckEnDis=on  GPIO_InputPcrCheckEnDis=on  eDMA_PcrCheckEnDis=on  PIT_PcrCheckEnDis=on  AMMCLIB_PcrCheckEnDis=on  FM_PcrCheckEnDis=on  Profiler_PcrCheckEnDis=on  ModelRef_PcrCheckEnDis=on  ModelPinCheck_PcrCheckEnDis=on
      | System Clock : 200 MHz
      | Target : MPC5744P
      | Package : 144LQFP
      | XTAL Freq : 40 MHz
      | Compiler : S32 Design Studio
      | Target Type : FLASH
      | Global Interrupt Priority : 8
      | System Tick Interrupt Priority : 12
      | Freemaster : None;
      | Download Code after build : off

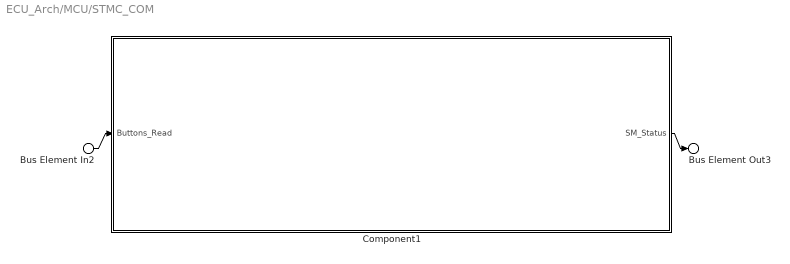
== system ECU_Arch/MCU/STMC_COM ==
  Bus Element In2 : Inport  PortName=Buttons_Read
  Component1 : Subsystem
      settings: PortSchema="{\"entries\":[{\"content\":{\"headerSize\":26,\"margin\":15,\"minimumSpacing\":25,\"sides\":[{\"content\":{\"connectorIds\":[\"In1\"]},\"type\":\"ConnectorPlacement.EquallySpacedRectSide\",\"uuid\":\"9e3c9234-344f-41fb-9145-1ecb76f9604b\"},{\"content\":{\"connectorIds\":[\"Out1\"],\"side\":\"RIGHT\"},\"type\":\"ConnectorPlacement.EquallySpacedRectSide\",\"uuid\":\"91314b46-0148-4d0b-8df6-e1be712fb317\"},{\"content\":{\"connectorIds\":[],\"side\":\"TOP\"},\"type\":\"ConnectorPlacement.EquallySpacedRectSide\",\"uuid\":\"6d51069f-a7df-430f-ba3a-6b16d510f018\"}]},\"type\":\"ConnectorPlacement.EquallySpacedConnector\",\"uuid\":\"067f1f1b-f809-4f0e-9eeb-c5481468f53e\"}],\"packageUris\":[\"http://schema.mathworks.com/mf0/Connector/R2020b\"],\"version\":\"1.0\"}"
  Bus Element Out3 : Outport  PortName=SM_Status
  wires:
  Bus Element In2/1 -> Component1/1(Buttons_Read)
  Component1/1(SM_Status) -> Bus Element Out3/1

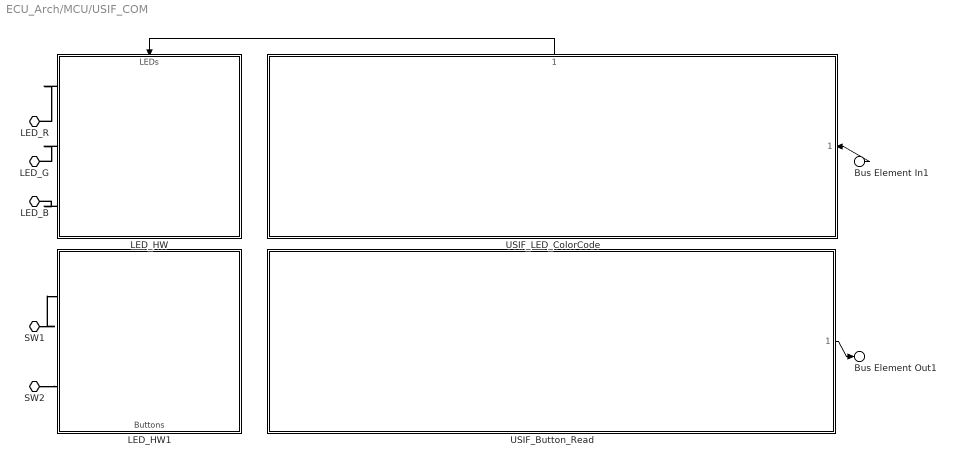
== system ECU_Arch/MCU/USIF_COM ==
  Bus Element In1 : Inport  PortName=SM_Status
  LED_HW : Subsystem
      settings: PortSchema="{\"entries\":[{\"content\":{\"headerSize\":26,\"margin\":15,\"minimumSpacing\":25,\"sides\":[{\"content\":{\"connectorIds\":[\"LConn1\",\"LConn2\",\"LConn3\"]},\"type\":\"ConnectorPlacement.EquallySpacedRectSide\",\"uuid\":\"86444d43-2102-435b-8a2b-2b030df31f7f\"},{\"content\":{\"connectorIds\":[],\"side\":\"RIGHT\"},\"type\":\"ConnectorPlacement.EquallySpacedRectSide\",\"uuid\":\"c9affe92-4cbe-435b-b672-be3201d83085\"},{\"content\":{\"connectorIds\":[\"In1\"],\"side\":\"TOP\"},\"type\":\"ConnectorPlacement.EquallySpacedRectSide\",\"uuid\":\"e6c64d0d-1c2e-4e7d-8b2e-cc6685d12efc\"}]},\"type\":\"ConnectorPlacement.EquallySpacedConnector\",\"uuid\":\"f562d7e9-72f8-4f82-93b3-f0475cfb8281\"}],\"packageUris\":[\"http://schema.mathworks.com/mf0/Connector/R2020b\"],\"version\":\"1.0\"}"
  LED_HW1 : Subsystem
      settings: PortSchema="{\"entries\":[{\"content\":{\"headerSize\":26,\"margin\":15,\"minimumSpacing\":25,\"sides\":[{\"content\":{\"connectorIds\":[\"LConn1\",\"LConn2\"]},\"type\":\"ConnectorPlacement.EquallySpacedRectSide\",\"uuid\":\"86444d43-2102-435b-8a2b-2b030df31f7f\"},{\"content\":{\"connectorIds\":[],\"side\":\"RIGHT\"},\"type\":\"ConnectorPlacement.EquallySpacedRectSide\",\"uuid\":\"c9affe92-4cbe-435b-b672-be3201d83085\"},{\"content\":{\"connectorIds\":[],\"side\":\"TOP\"},\"type\":\"ConnectorPlacement.EquallySpacedRectSide\",\"uuid\":\"e6c64d0d-1c2e-4e7d-8b2e-cc6685d12efc\"},{\"content\":{\"connectorIds\":[\"Out1\"],\"side\":\"BOTTOM\"},\"type\":\"ConnectorPlacement.EquallySpacedRectSide\",\"uuid\":\"fb853ae8-c8ba-4509-97c6-d7c02568cc68\"}]},\"type\":\"ConnectorPlacement.EquallySpacedConnector\",\"uuid\":\"f562d7e9-72f8-4f82-93b3-f0475cfb8281\"}],\"packageUris\":[\"http://schema.mathworks.com/mf0/Connector/R2020b\"],\"version\":\"1.0\"}"
  USIF_Button_Read : Subsystem  ReferencedSubsystem=USIF_Button_Read
      settings: PortSchema="{\"entries\":[{\"content\":{\"headerSize\":26,\"margin\":15,\"minimumSpacing\":25,\"sides\":[{\"content\":{\"connectorIds\":[]},\"type\":\"ConnectorPlacement.EquallySpacedRectSide\",\"uuid\":\"86444d43-2102-435b-8a2b-2b030df31f7f\"},{\"content\":{\"connectorIds\":[\"Out1\"],\"side\":\"RIGHT\"},\"type\":\"ConnectorPlacement.EquallySpacedRectSide\",\"uuid\":\"c9affe92-4cbe-435b-b672-be3201d83085\"},{\"content\":{\"connectorIds\":[],\"side\":\"TOP\"},\"type\":\"ConnectorPlacement.EquallySpacedRectSide\",\"uuid\":\"e6c64d0d-1c2e-4e7d-8b2e-cc6685d12efc\"},{\"content\":{\"connectorIds\":[],\"side\":\"BOTTOM\"},\"type\":\"ConnectorPlacement.EquallySpacedRectSide\",\"uuid\":\"8223df01-dc71-484a-b29a-5f5baa25ea41\"}]},\"type\":\"ConnectorPlacement.EquallySpacedConnector\",\"uuid\":\"f562d7e9-72f8-4f82-93b3-f0475cfb8281\"}],\"packageUris\":[\"http://schema.mathworks.com/mf0/Connector/R2020b\"],\"version\":\"1.0\"}"
  USIF_LED_ColorCode : Subsystem  ReferencedSubsystem=USIF_LED_ColorCode
      settings: PortSchema="{\"entries\":[{\"content\":{\"headerSize\":26,\"margin\":15,\"minimumSpacing\":25,\"sides\":[{\"content\":{\"connectorIds\":[]},\"type\":\"ConnectorPlacement.EquallySpacedRectSide\",\"uuid\":\"86444d43-2102-435b-8a2b-2b030df31f7f\"},{\"content\":{\"connectorIds\":[\"In1\"],\"side\":\"RIGHT\"},\"type\":\"ConnectorPlacement.EquallySpacedRectSide\",\"uuid\":\"c9affe92-4cbe-435b-b672-be3201d83085\"},{\"content\":{\"connectorIds\":[\"Out1\"],\"side\":\"TOP\"},\"type\":\"ConnectorPlacement.EquallySpacedRectSide\",\"uuid\":\"e6c64d0d-1c2e-4e7d-8b2e-cc6685d12efc\"}]},\"type\":\"ConnectorPlacement.EquallySpacedConnector\",\"uuid\":\"f562d7e9-72f8-4f82-93b3-f0475cfb8281\"}],\"packageUris\":[\"http://schema.mathworks.com/mf0/Connector/R2020b\"],\"version\":\"1.0\"}"
  SW1 : PMIOPort  Side=Left
  SW2 : PMIOPort  Port=2  Side=Left
  LED_R : PMIOPort  Port=3  Side=Left
  LED_G : PMIOPort  Port=4  Side=Left
  LED_B : PMIOPort  Port=5  Side=Left
  Bus Element Out1 : Outport  PortName=Buttons_Read
  wires:
  Bus Element In1/1 -> USIF_LED_ColorCode/1
  USIF_Button_Read/1 -> Bus Element Out1/1
  USIF_LED_ColorCode/1 -> LED_HW/1(LEDs)
  connections:
  LED_HW/LConn3 -- LED_B/RConn1
  LED_HW/LConn2 -- LED_G/RConn1
  LED_HW/LConn1 -- LED_R/RConn1
  SW1/RConn1 -- LED_HW1/LConn1
  SW2/RConn1 -- LED_HW1/LConn2

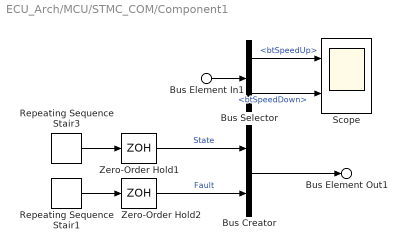
== system ECU_Arch/MCU/STMC_COM/Component1 ==
  Bus Element In1 : Inport  PortName=Buttons_Read
  Bus Creator : BusCreator  Inputs=2
  Bus Selector : BusSelector  OutputSignals=btSpeedUp,btSpeedDown
  Repeating Sequence Stair1 : simulink/Sources/Repeating Sequence Stair  OutValues=[0 1].'  tsamp=-1  OutMin=[]  OutMax=[]  OutDataTypeStr=uint8  OutputDataTypeScalingMode=uint8  OutDataType=fixdt(0,8)  ConRadixGroup=Best Precision: Vector-wise  OutScaling=2^-12
  Repeating Sequence Stair3 : simulink/Sources/Repeating Sequence Stair  OutValues=[0 1].'  tsamp=-1  OutMin=[]  OutMax=[]  OutDataTypeStr=uint8  OutputDataTypeScalingMode=uint8  OutDataType=fixdt(0,8)  ConRadixGroup=Best Precision: Vector-wise  OutScaling=2^-12
  Scope : Scope  NumInputPorts=2
  Zero-Order Hold1 : ZeroOrderHold  SampleTime=0.1
  Zero-Order Hold2 : ZeroOrderHold  SampleTime=0.1
  Bus Element Out1 : Outport  PortName=SM_Status
  wires:
  Bus Element In1/1 -> Bus Selector/1
  Bus Selector/1 -> Scope/1  "<btSpeedUp>"
  Bus Selector/2 -> Scope/2  "<btSpeedDown>"
  Bus Creator/1 -> Bus Element Out1/1
  Repeating Sequence Stair1/1 -> Zero-Order Hold2/1
  Repeating Sequence Stair3/1 -> Zero-Order Hold1/1
  Zero-Order Hold1/1 -> Bus Creator/1  "State"
  Zero-Order Hold2/1 -> Bus Creator/2  "Fault"

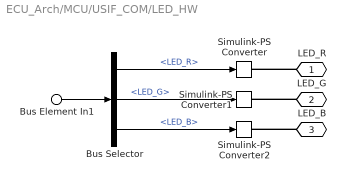
== system ECU_Arch/MCU/USIF_COM/LED_HW ==
  Bus Element In1 : Inport  PortName=LEDs
  Bus Selector : BusSelector  OutputSignals=LED_R,LED_G,LED_B
  Simulink-PS Converter : nesl_utility/Simulink-PS Converter  PhysicalDomain=network_engine_domain  SubClassName=ps_input  LeftPortType=input  RightPortType=output  PseudoPeriodic=off  Frequencies=[]  NoiseDistribution=none  NoiseParameters=[]  Unit=1  AffineConversion=off  FilteringAndDerivatives=provide  SimscapeFilterOrder=1  InputFilterTimeConstant=0.001  UdotUserProvided=0
  Simulink-PS Converter1 : nesl_utility/Simulink-PS Converter  PhysicalDomain=network_engine_domain  SubClassName=ps_input  LeftPortType=input  RightPortType=output  PseudoPeriodic=off  Frequencies=[]  NoiseDistribution=none  NoiseParameters=[]  Unit=1  AffineConversion=off  FilteringAndDerivatives=provide  SimscapeFilterOrder=1  InputFilterTimeConstant=0.001  UdotUserProvided=0
  Simulink-PS Converter2 : nesl_utility/Simulink-PS Converter  PhysicalDomain=network_engine_domain  SubClassName=ps_input  LeftPortType=input  RightPortType=output  PseudoPeriodic=off  Frequencies=[]  NoiseDistribution=none  NoiseParameters=[]  Unit=1  AffineConversion=off  FilteringAndDerivatives=provide  SimscapeFilterOrder=1  InputFilterTimeConstant=0.001  UdotUserProvided=0
  LED_R : PMIOPort  Side=Left
  LED_G : PMIOPort  Port=2  Side=Left
  LED_B : PMIOPort  Port=3  Side=Left
  wires:
  Bus Element In1/1 -> Bus Selector/1
  Bus Selector/1 -> Simulink-PS Converter/1  "<LED_R>"
  Bus Selector/2 -> Simulink-PS Converter1/1  "<LED_G>"
  Bus Selector/3 -> Simulink-PS Converter2/1  "<LED_B>"
  connections:
  LED_R/RConn1 -- Simulink-PS Converter/RConn1
  LED_G/RConn1 -- Simulink-PS Converter1/RConn1
  LED_B/RConn1 -- Simulink-PS Converter2/RConn1

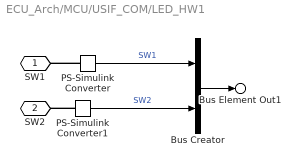
== system ECU_Arch/MCU/USIF_COM/LED_HW1 ==
  Bus Creator : BusCreator  Inputs=2
  PS-Simulink Converter : nesl_utility/PS-Simulink Converter  PhysicalDomain=network_engine_domain  SubClassName=ps_output  LeftPortType=input  RightPortType=output  PseudoPeriodic=off  Frequencies=[]  VectorFormat=inherit  Unit=inherit  AffineConversion=off
  PS-Simulink Converter1 : nesl_utility/PS-Simulink Converter  PhysicalDomain=network_engine_domain  SubClassName=ps_output  LeftPortType=input  RightPortType=output  PseudoPeriodic=off  Frequencies=[]  VectorFormat=inherit  Unit=inherit  AffineConversion=off
  SW1 : PMIOPort  Side=Left
  SW2 : PMIOPort  Port=2  Side=Left
  Bus Element Out1 : Outport  PortName=Buttons
  wires:
  PS-Simulink Converter/1 -> Bus Creator/1  "SW1"
  PS-Simulink Converter1/1 -> Bus Creator/2  "SW2"
  Bus Creator/1 -> Bus Element Out1/1
  connections:
  PS-Simulink Converter/LConn1 -- SW1/RConn1
  PS-Simulink Converter1/LConn1 -- SW2/RConn1
